simulink library "bach_library"  (R2020b)
settings: Solver=VariableStepAuto  StartTime=0.0  StopTime=10.0  RelTol=1e-3
settings Model: Creator=martin  LastModifiedBy=Martin

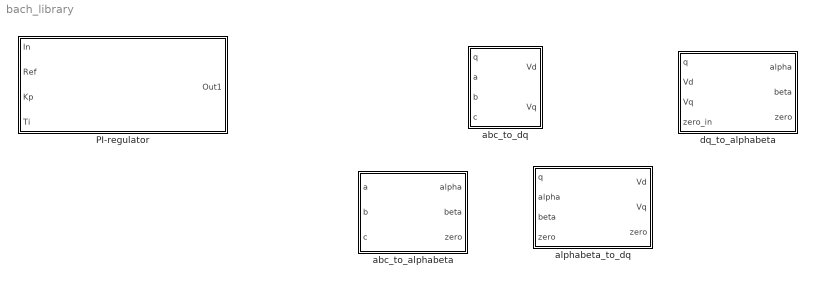
== system bach_library ==
  PI-regulator : Subsystem
  abc_to_alphabeta : MATLAB Function  TreatAsAtomicUnit=on
  abc_to_dq : MATLAB Function  TreatAsAtomicUnit=on
  alphabeta_to_dq : MATLAB Function  TreatAsAtomicUnit=on
  dq_to_alphabeta : MATLAB Function  TreatAsAtomicUnit=on

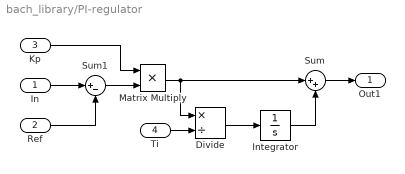
== system bach_library/PI-regulator ==
  In : Inport
  Ref : Inport  Port=2
  Kp : Inport  Port=3
  Ti : Inport  Port=4
  Divide : Product  Inputs=*/
  Integrator : Integrator
  Matrix Multiply : Product
  Sum : Sum  Inputs=|++
  Sum1 : Sum  Inputs=|+-
  Out1 : Outport
  wires:
  Matrix Multiply/1 -> Sum/1, Divide/1
  Integrator/1 -> Sum/2
  Divide/1 -> Integrator/1
  Sum1/1 -> Matrix Multiply/2
  In/1 -> Sum1/1
  Ref/1 -> Sum1/2
  Kp/1 -> Matrix Multiply/1
  Ti/1 -> Divide/2
  Sum/1 -> Out1/1

== matlab function bach_library/dq_to_alphabeta ==
  data: q input; alpha output; Vd input; Vq input; zero_in input; beta output; zero output
function [alpha, beta, zero] = dq_to_alphabeta(q, Vd, Vq, zero_in)

Vab = [cos(q) -sin(q) 0;sin(q) cos(q) 0;0 0 1]*[Vd; Vq; zero_in];
alpha = Vab(1,:);
beta = Vab(2,:);
zero = Vab(3,:);

== matlab function bach_library/abc_to_dq ==
  data: Vd output; q input; a input; Vq output; b input; c input
function [Vd,Vq] = abc_to_dq(q, a, b, c)

% 2/3 in stead of sqrt(2/3)!

Vabc = [a;b;c];
Vdq = 2/3*[cos(q) cos(q-2*pi/3) cos(q+2*pi/3); 
     -sin(q) -sin(q-2*pi/3) -sin(q+2*pi/3)] * Vabc;

Vd = Vdq(1,:);
Vq = Vdq(2,:);

== matlab function bach_library/abc_to_alphabeta ==
  data: alpha output; a input; beta output; b input; c input; zero output
function [alpha, beta, zero] = abc_to_alphabeta(a, b, c)

% 2/3 in stead of sqrt(2/3)!
Valphabeta = 2/3*[1         -1/2        -1/2;
                  0         sqrt(3)/2   -sqrt(3)/2;
                  1/2       1/2         1/2]      * [a;b;c];

alpha = Valphabeta(1,:);
beta = Valphabeta(2,:);
zero = Valphabeta(3,:);

== matlab function bach_library/alphabeta_to_dq ==
  data: Vd output; q input; alpha input; beta input; zero input; Vq output; zero output
function [Vd, Vq, zero] = alphabeta_to_dq(q, alpha, beta, zero)

Vdq = [cos(q) sin(q) 0;-sin(q) cos(q) 0;0 0 1]*[alpha;beta;zero];
Vd = Vdq(1,:);
Vq = Vdq(2,:);
zero = Vdq(3,:);
